simulink model "Graphical_Func_Calc"  (R2016a)
settings: Solver=VariableStepAuto  StartTime=0.0  StopTime=10.0  RelTol=1e-3
settings Model: Creator=LEGION  LastModifiedBy=LEGION

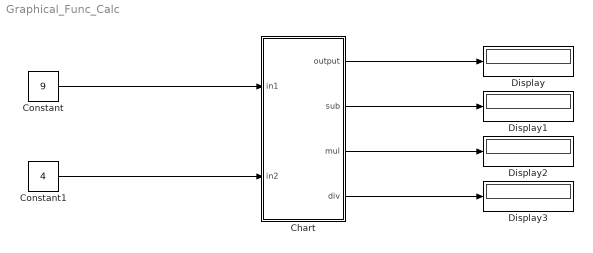
== system Graphical_Func_Calc ==
  Chart : Stateflow chart  TreatAsAtomicUnit=on
  Constant : Constant  Value=9
  Constant1 : Constant  Value=4
  Display{,1..3} (4 alike) : Display
  wires:
  Constant/1 -> Chart/1(in1)
  Constant1/1 -> Chart/2(in2)
  Chart/1(output) -> Display/1
  Chart/2(sub) -> Display1/1
  Chart/3(mul) -> Display2/1
  Chart/4(div) -> Display3/1

== stateflow chart Graphical_Func_Calc/Chart ==
  state out = DIV(op1,op2) [function]
    (default) -> (junction 41) : {out = op2/op1}
  state out = MUL(op1,op2) [function]
    (default) -> (junction 49) : {out = op2 * op1}
  state out = ADD(op1,op2) [function]
    (default) -> (junction 17) : {out = op1+op2}
  state out = SUB(op1,op2) [function]
    (default) -> (junction 26) : {out = op2 - op1}
  (default) -> (junction 43) : {div = DIV(in1,in2)
      |
      | mul = MUL(in1,in2)
      | output = ADD(in1,in2)
      |
      | sub = SUB(in1,in2)
      |
      | }
  data: op1 function_input; op2 function_input; out function_output; op1 function_input; op2 function_input; out function_output; op1 function_input; op2 function_input; out function_output; op1 function_input; op2 function_input; out function_output; in1 input; in2 input; output output; sub output; mul output; div output
